simulink model "topiir"  (Simulink 6.3)
settings: Solver=FixedStepDiscrete  StartTime=0.0  StopTime=100  RelTol=1e-3
PreLoadFcn:
  | topiirinit
InitFcn:
  | %% DSPBuilder Start
  | alt_dspbuilder_update_model(bdroot)
  | %% DSPBuilder End
undefined symbols (not defined in the file or in its folder): Den, Num
libraries: allblocks_alteradspbuilder2 x14
settings Model: Creator=mjervis  LastModifiedBy=LKONG
settings DataIOCC: SignalLoggingName=sigsOut
settings OptimizationCC: BooleanDataType=off  InlineInvariantSignals=on
settings DebuggingCC: SolverPrmCheckMsg=none
settings HardwareCC: TargetUnknown=on

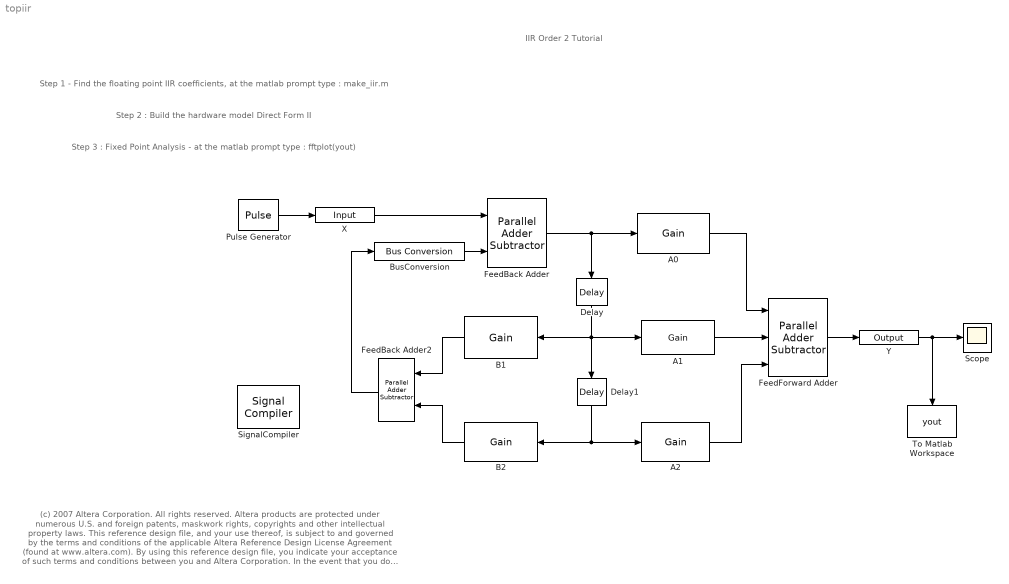
== system topiir ==
  note: Step 1 - Find the floating point IIR coefficients, at the matlab prompt type : make_iir.m
  note: Step 3 : Fixed Point Analysis - at the matlab prompt type : fftplot(yout)
  note: IIR Order 2 Tutorial
  note: Step 2 : Build the hardware model Direct Form II
  note: (c) 2007 Altera Corporation. All rights reserved.  Altera products are protected under numerous U.S. and foreign patents, maskwork rights, copyrights and other intellectual property laws.
      | This reference design file, and your use thereof, is subject to and governed by the terms and conditions of the applicable Altera Reference Design License Agreement (found at www.altera.com).
      | By using this reference design file, you indicate your acceptance of such terms and conditions between you and Altera Corporation.
      | In the event that you do not agree with such terms and conditions, you may not use the reference design file and please promptly destroy any copies you have made.
      | This reference design file being provided on an "as-is" basis and as an accommodation and therefore all warranties, representations or guarantees of any kind (whether express, implied or statutory)
      | including, without limitation, warranties of merchantability, non-infringement, or fitness for a particular purpose, are specifically disclaimed.
      | By making this reference design file available, Altera expressly does not recommend, suggest or require that this reference design file be used in combination with any other product not provided by Altera
  A0 : allblocks_alteradspbuilder2/Gain  vgain=Num(1)  BusType=Signed Fractional  bwl=2  bwr=12  pipeline=0  use_ena=off  use_aclr=off  lpm=off  MaskValue=1
  A1 : allblocks_alteradspbuilder2/Gain  vgain=Num(2)  BusType=Signed Fractional  bwl=2  bwr=12  pipeline=0  use_ena=off  use_aclr=off  lpm=off  MaskValue=1
  A2 : allblocks_alteradspbuilder2/Gain  vgain=Num(3)  BusType=Signed Fractional  bwl=2  bwr=12  pipeline=0  use_ena=off  use_aclr=off  lpm=off  MaskValue=1
  B1 : allblocks_alteradspbuilder2/Gain  Orientation=left  vgain=Den(2)  BusType=Signed Fractional  bwl=2  bwr=12  pipeline=0  use_ena=off  use_aclr=off  lpm=off  MaskValue=1
  B2 : allblocks_alteradspbuilder2/Gain  Orientation=left  vgain=Den(3)  BusType=Signed Fractional  bwl=2  bwr=12  pipeline=0  use_ena=off  use_aclr=off  lpm=off  MaskValue=1
  BusConversion : allblocks_alteradspbuilder2/Bus Conversion  BusType=Signed Fractional  ibwl=5  ibwr=21  bwl=2  bwr=8  bitToConnectToOutputLSB=3  round=off  saturate=off
  Delay : allblocks_alteradspbuilder2/Delay  Orientation=down  pipeline=1  ClockPhase=1  use_ena=off  use_sclr=off
  Delay1 : allblocks_alteradspbuilder2/Delay  Orientation=down  pipeline=1  ClockPhase=1  use_ena=off  use_sclr=off
  FeedBack Adder : allblocks_alteradspbuilder2/Parallel Adder Subtractor  number_of_inputs=2  direction=++  use_pipeline=off  phase_selection=1  use_ena=off  use_aclr=off
  FeedBack Adder2 : allblocks_alteradspbuilder2/Parallel Adder Subtractor  Orientation=left  number_of_inputs=2  direction=++  use_pipeline=off  phase_selection=1  use_ena=off  use_aclr=off
  FeedForward Adder : allblocks_alteradspbuilder2/Parallel Adder Subtractor  number_of_inputs=3  direction=++  use_pipeline=off  phase_selection=1  use_ena=off  use_aclr=off
  Pulse Generator : DiscretePulseGenerator  Period=2000  PhaseDelay=3
  Scope : Scope
      settings: TimeRange=100  YMin=-0.1  YMax=0.4
  SignalCompiler : allblocks_alteradspbuilder2/Signal Compiler  DeviceFamily=Cyclone III  DeviceName=AUTO  EnableSignalTap=off  SignalTapDepth=128  UseBoardBlock=off  StpUseDefaultClock=on  StpClock=Clock
  To Matlab Workspace : ToWorkspace  VariableName=yout  SampleTime=-1  SaveFormat=Array
      settings: Orientation=down
  X : allblocks_alteradspbuilder2/Input  iofile=d:\workspace\Documentation\DesignExamples\Demos\Filters\IIROrder2\tb_topiir\topiir_X.salt  BusType=Signed Fractional  bwl=2  bwr=8  SpecifyClock=off  PORTTYPE=Input
  Y : allblocks_alteradspbuilder2/Output  iofile=d:\workspace\Documentation\DesignExamples\Demos\Filters\IIROrder2\tb_topiir\topiir_Y.capture  BusType=Signed Fractional  bwl=4  bwr=12  PORTTYPE=Output
  wires:
  Delay/1 -> A1/1, Delay1/1, B1/1
  FeedBack Adder/1 -> Delay/1, A0/1
  BusConversion/1 -> FeedBack Adder/2
  A0/1 -> FeedForward Adder/1
  A1/1 -> FeedForward Adder/2
  X/1 -> FeedBack Adder/1
  FeedForward Adder/1 -> Y/1
  Y/1 -> Scope/1, To Matlab Workspace/1
  Delay1/1 -> B2/1, A2/1
  A2/1 -> FeedForward Adder/3
  B1/1 -> FeedBack Adder2/1
  B2/1 -> FeedBack Adder2/2
  FeedBack Adder2/1 -> BusConversion/1
  Pulse Generator/1 -> X/1
